simulink model "Sim50"  (R2019a)
settings: Solver=FixedStepAuto  StartTime=0.0  StopTime=10.0  FixedStep=0.0001  RelTol=1e-3
settings Model: Creator=fbleo  LastModifiedBy=fbleo

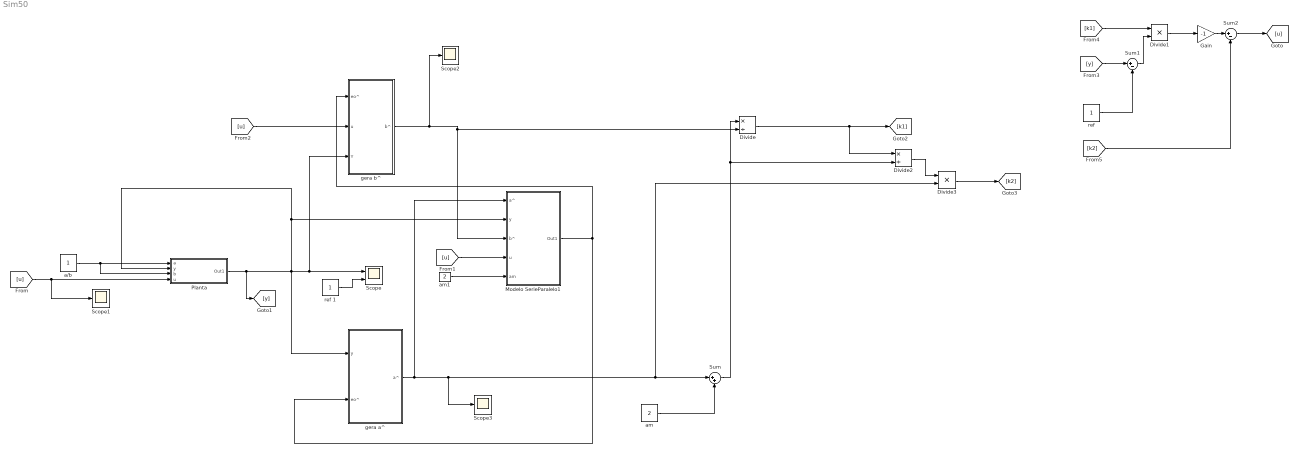
== system Sim50 ==
  Divide : Product  Inputs=*/
  Divide1 : Product  Inputs=**
  Divide2 : Product  Inputs=*/
  Divide3 : Product  Inputs=**
  Gain : Gain  Gain=-1
  Modelo SerieParalelo1 : Subsystem
  Planta : Subsystem
  Scope : Scope  NumInputPorts=2
  Scope1 : Scope
  Scope2 : Scope
  Scope3 : Scope
  Sum : Sum  Inputs=|++
  Sum1 : Sum  Inputs=|+-
  Sum2 : Sum  Inputs=|+-
  a/b : Constant
  am : Constant  Value=2
  am1 : Constant  Value=2
  gera a^ : Subsystem
  gera b^ : Subsystem
  ref : Constant
  ref 1 : Constant
  wires:
  Planta/1(Out1) -> [y], gera a^/1(y), Planta/2(y), Modelo SerieParalelo1/2(y), gera b^/3("Y "), Scope/1
  Modelo SerieParalelo1/1(Out1) -> gera b^/1(eo^), gera a^/2(eo^)
  Sum/1 -> Divide2/2, Divide/1
  [u] -> Modelo SerieParalelo1/4(u)
  [u] -> Scope1/1, Planta/4(u)
  a/b/1 -> Planta/3(b), Planta/1(a)
  am1/1 -> Modelo SerieParalelo1/5(am)
  gera a^/1(a^) -> Modelo SerieParalelo1/1(a^), Scope3/1, Divide3/2, Sum/1
  am/1 -> Sum/2
  [u] -> gera b^/2(u)
  Sum1/1 -> Divide1/2
  Divide/1 -> Divide2/1, [k1]
  Divide1/1 -> Gain/1
  [k2] -> Sum2/2
  [y] -> Sum1/1
  Gain/1 -> Sum2/1
  Sum2/1 -> [u]
  [k1] -> Divide1/1
  Divide3/1 -> [k2]
  ref/1 -> Sum1/2
  gera b^/1(b^) -> Scope2/1, Divide/2, Modelo SerieParalelo1/3(b^)
  Divide2/1 -> Divide3/1
  ref 1/1 -> Scope/2

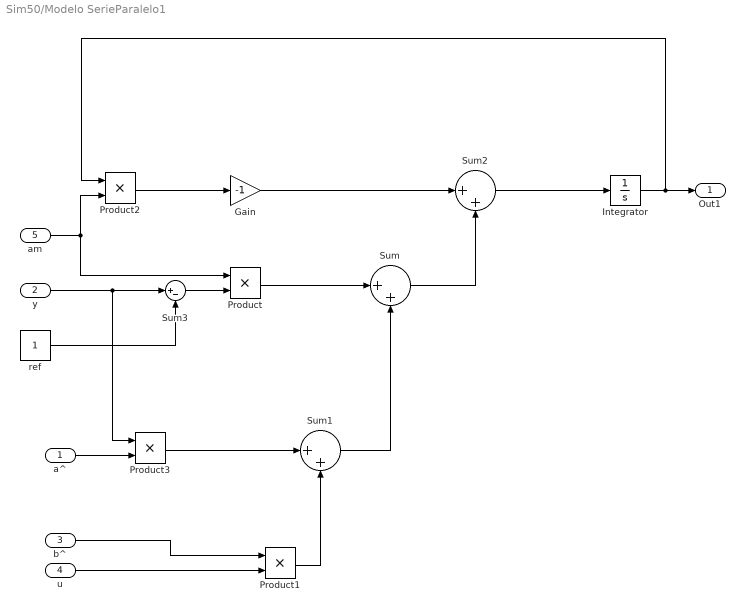
== system Sim50/Modelo SerieParalelo1 ==
  a^ : Inport
  y : Inport  Port=2
  b^ : Inport  Port=3
  u : Inport  Port=4
  am : Inport  Port=5
  Gain : Gain  Gain=-1
  Integrator : Integrator  InitialCondition=1.25
  Product{,1..3} (4 alike) : Product
  Sum : Sum  Inputs=|++
  Sum1 : Sum  Inputs=|++
  Sum2 : Sum  Inputs=|++
  Sum3 : Sum  Inputs=|+-
  ref : Constant
  Out1 : Outport
  wires:
  Product/1 -> Sum/1
  u/1 -> Product1/2
  b^/1 -> Product1/1
  Product1/1 -> Sum1/2
  Sum/1 -> Sum2/2
  Integrator/1 -> Product2/1, Out1/1
  am/1 -> Product/1, Product2/2
  Product2/1 -> Gain/1
  Gain/1 -> Sum2/1
  Sum2/1 -> Integrator/1
  ref/1 -> Sum3/2
  y/1 -> Product3/1, Sum3/1
  Sum3/1 -> Product/2
  a^/1 -> Product3/2
  Product3/1 -> Sum1/1
  Sum1/1 -> Sum/2

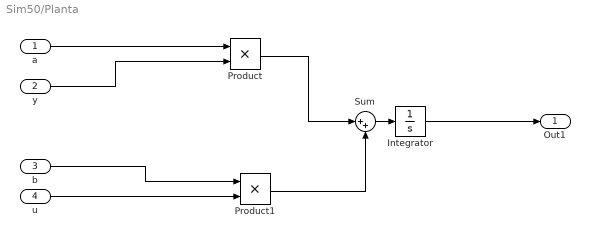
== system Sim50/Planta ==
  a : Inport
  y : Inport  Port=2
  b : Inport  Port=3
  u : Inport  Port=4
  Integrator : Integrator  InitialCondition=0.5
  Product : Product
  Product1 : Product
  Sum : Sum  Inputs=|++
  Out1 : Outport
  wires:
  a/1 -> Product/1
  y/1 -> Product/2
  Product/1 -> Sum/1
  u/1 -> Product1/2
  b/1 -> Product1/1
  Product1/1 -> Sum/2
  Sum/1 -> Integrator/1
  Integrator/1 -> Out1/1

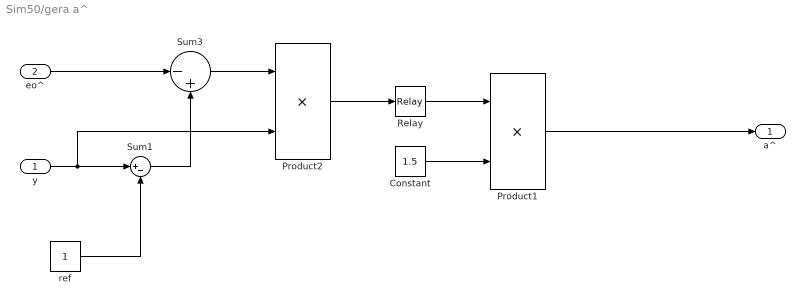
== system Sim50/gera a^ ==
  y : Inport
  eo^ : Inport  Port=2
  Constant : Constant  Value=1.5
  Product1 : Product
  Product2 : Product
  Relay : Relay  OnSwitchValue=0.01  OffSwitchValue=-0.01  OffOutputValue=-1
  Sum1 : Sum  Inputs=|+-
  Sum3 : Sum  Inputs=|-+
  ref : Constant
  a^ : Outport
  wires:
  Sum3/1 -> Product2/1
  eo^/1 -> Sum3/1
  Product1/1 -> a^/1
  Product2/1 -> Relay/1
  Relay/1 -> Product1/1
  Constant/1 -> Product1/2
  ref/1 -> Sum1/2
  y/1 -> Product2/2, Sum1/1
  Sum1/1 -> Sum3/2

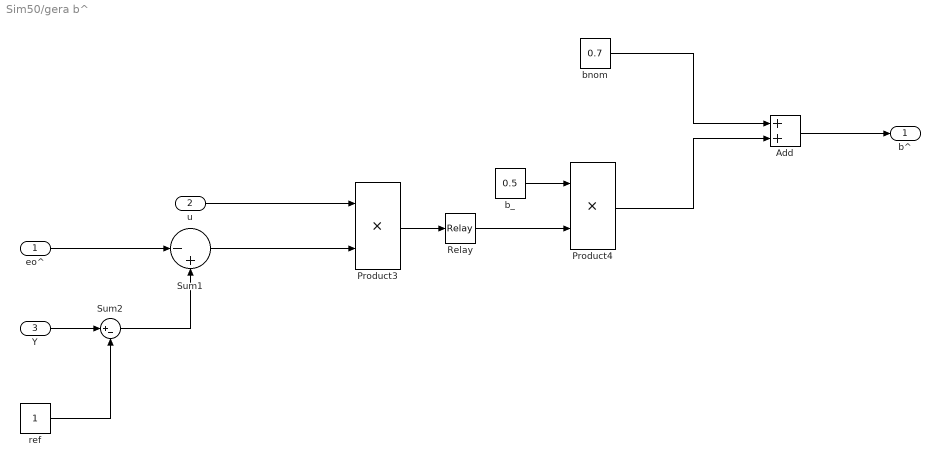
== system Sim50/gera b^ ==
  eo^ : Inport
  u : Inport  Port=2
  "Y " : Inport  Port=3
  Add : Sum
  Product3 : Product
  Product4 : Product
  Relay : Relay  OnSwitchValue=0.01  OffSwitchValue=-0.01  OffOutputValue=-1
  Sum1 : Sum  Inputs=|-+
  Sum2 : Sum  Inputs=|+-
  b_ : Constant  Value=0.5
  bnom : Constant  Value=0.7
  ref : Constant
  b^ : Outport
  wires:
  u/1 -> Product3/1
  eo^/1 -> Sum1/1
  Sum1/1 -> Product3/2
  Product3/1 -> Relay/1
  b_/1 -> Product4/1
  bnom/1 -> Add/1
  Product4/1 -> Add/2
  Relay/1 -> Product4/2
  ref/1 -> Sum2/2
  "Y "/1 -> Sum2/1
  Sum2/1 -> Sum1/2
  Add/1 -> b^/1
